simulink model "lab6"  (R2023b)
settings: Solver=ode45  StartTime=0.0  StopTime=50.0  MaxStep=2^(-5)  RelTol=1e-3
settings Model: Creator=insomnia  LastModifiedBy=insomnia

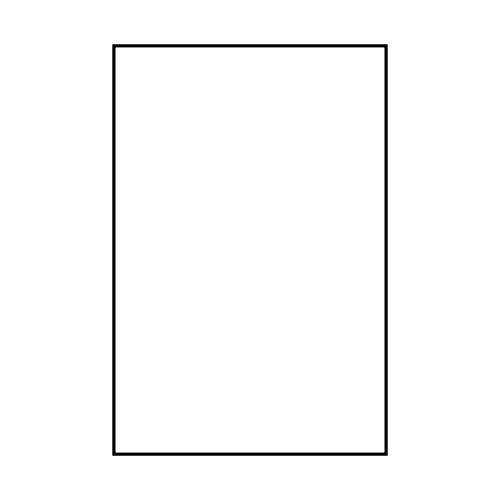
[thumbnail: Simulink's stored preview of the top-level diagram]
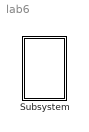
== system lab6 ==
  Subsystem : Subsystem  mask{g=9.81, m1=1, m2=3, M=1, R=0.001, r0=1, r1=0, th0=90, th1=0}
      mask prompts: g "przyspieszenie ziemskie"; m1 "masa wahadla"; m2 "masa ciezarka"; M "masa bloczkow"; R "promien bloczkow"; r0 "poczatkowa dlugosc linki"; r1 "zapomniane r1"; th0 "poczatkowy kat"; th1 "zapomniane th1"

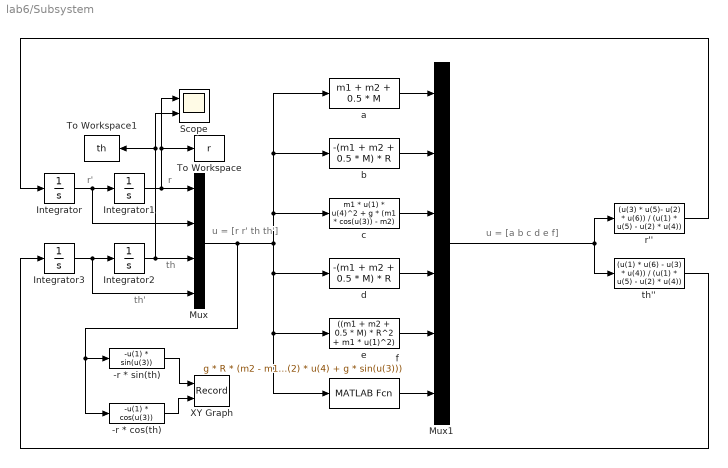
== system lab6/Subsystem ==
  note: u = [a b c d e f]
  note: th
  note: th'
  note: r'
  note: r
  note: u = [r r' th th']
  -r * cos(th) : MATLABFcn  MATLABFcn=-u(1) * cos(u(3))
  -r * sin(th) : MATLABFcn  MATLABFcn=-u(1) * sin(u(3))
  Integrator : Integrator  InitialCondition=r1
  Integrator1 : Integrator  InitialCondition=r0
  Integrator2 : Integrator  InitialCondition=th0 * pi / 180
  Integrator3 : Integrator  InitialCondition=th1 * pi / 180
  Mux : Mux
  Mux1 : Mux  Inputs=6
  Scope : Scope  NumInputPorts=2
  To Workspace : ToWorkspace  VariableName=r  SampleTime=-1
  To Workspace1 : ToWorkspace  VariableName=th  SampleTime=-1
  XY Graph : Record  FileSettingsInternal="{\"entries\":[{\"content\":{\"excelSettings\":{\"content\":{},\"type\":\"Streamout.ExcelSettings\"}},\"type\":\"Streamout.FileSettingStorage\",\"uuid\":\"\"}],\"packageUris\":[\"http:\\/\\/schema.mathworks.com\\/mf0\\/streamout_blocks\\/R2020a\"],\"version\":\"1.0\"}"  Layout=[1 1]  SignalsInternal="{\"entries\":[{\"content\":{\"signals\":[{\"content\":{\"blockPath\":[],\"dimensions\":[1],\"domain\":\"\",\"lineColor\":\"#a2142f\",\"plots\":[ 1 ],\"port\":1,\"signalID\":1,\"signalName\":\"-r * sin(th)\"},\"type\":\"RecordBlkView.Signal\",\"uuid\":\"\"},{\"content\":{\"blockPath\":[],\"dimensions\":[1],\"domain\":\"\",\"lineColor\":\"#139fff\",\"plots\":[ 1 ],\"port\":2,\"signalID\":2,\"signalName\":\"-r * cos(th)\"},\"type\":\"RecordBlkView.Signal\",\"uuid\":\"\"}]},\"type\":\"RecordBlkView.InputSignals\",\"uuid\":\"\"}],\"packageUris\":[\"http:\\/\\/schema.mathworks.com\\/mf0\\/streamout_blocks\\/R2020a\"],\"version\":\"1.0\"}"  VisualizationBindings="{\"xyplotplugin\":{\"info\":[{\"series\":[{\"bindingParametersList\":[{\"parameter\":\"X-Axis\",\"signalID\":1,\"signalName\":\"-r * sin(th)\"},{\"parameter\":\"Y-Axis\",\"signalID\":2,\"signalName\":\"-r * cos(th)\"}],\"seriesID\":0}],\"subplotID\":1}]}}"  CompatibilityTag=XY
  a : MATLABFcn  MATLABFcn=m1 + m2 + 0.5 * M
  b : MATLABFcn  MATLABFcn=-(m1 + m2 + 0.5 * M) * R
  c : MATLABFcn  MATLABFcn=m1 * u(1) * u(4)^2 + g * (m1 * cos(u(3)) - m2)
  d : MATLABFcn  MATLABFcn=-(m1 + m2 + 0.5 * M) * R
  e : MATLABFcn  MATLABFcn=((m1 + m2 + 0.5 * M) * R^2 + m1 * u(1)^2)
  f : MATLABFcn  MATLABFcn=g * R * (m2 - m1 * cos(u(3))) - m1 * u(1) * (2 * u(2) * u(4) + g * sin(u(3)))
  r'' : MATLABFcn  MATLABFcn=(u(3) * u(5)- u(2) * u(6)) / (u(1) * u(5) - u(2) * u(4))
  th'' : MATLABFcn  MATLABFcn=(u(1) * u(6) - u(3) * u(4)) / (u(1) * u(5) - u(2) * u(4))
  wires:
  a/1 -> Mux1/1
  th''/1 -> Integrator3/1
  Integrator3/1 -> Mux/4, Integrator2/1
  Mux/1 -> -r * cos(th)/1, -r * sin(th)/1, a/1, b/1, c/1, f/1, e/1, d/1
  Integrator/1 -> Mux/2, Integrator1/1
  c/1 -> Mux1/3
  Mux1/1 -> r''/1, th''/1
  f/1 -> Mux1/6
  b/1 -> Mux1/2
  r''/1 -> Integrator/1
  Integrator1/1 -> To Workspace/1, Scope/1, Mux/1
  e/1 -> Mux1/5
  d/1 -> Mux1/4
  Integrator2/1 -> To Workspace1/1, Scope/2, Mux/3
  -r * sin(th)/1 -> XY Graph/1
  -r * cos(th)/1 -> XY Graph/2
